simulink model "gradijentni_model"  (R2025a)
settings: Solver=VariableStepAuto  StartTime=0.0  StopTime=100  RelTol=1e-3
values from neighbouring files (symbols this model uses):
  Tf = 1    [mse.m]
settings Model: Creator=neso  LastModifiedBy=Korisnik

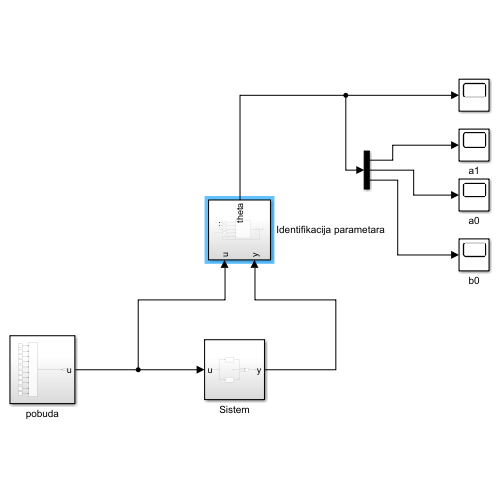
[thumbnail: Simulink's stored preview of the top-level diagram]
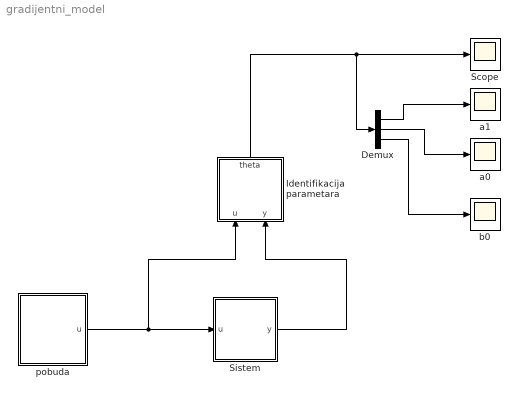
== system gradijentni_model ==
  Demux : Demux  Outputs=3
  Identifikacija parametara : Subsystem
  Scope : Scope
      settings: ActiveDisplayYMinimum=-10.408087644421066  ActiveDisplayYMaximum=16.003973276470475
  Sistem : Subsystem
  a0 : Scope
      settings: ActiveDisplayYMinimum=-8.5109294559908086  ActiveDisplayYMaximum=21.084373521888086  DataLoggingVariableName=ScopeData2
  a1 : Scope
      settings: ActiveDisplayYMinimum=0.935675841003011  ActiveDisplayYMaximum=9.3006227399808985
  b0 : Scope
      settings: ActiveDisplayYMinimum=-8.5109294559908086  ActiveDisplayYMaximum=21.084373521888086  DataLoggingVariableName=ScopeData3
  pobuda : Subsystem
  wires:
  Sistem/1(y) -> Identifikacija parametara/2(y)
  Identifikacija parametara/1(theta) -> Demux/1, Scope/1
  pobuda/1(u) -> Identifikacija parametara/1(u), Sistem/1(u)
  Demux/1 -> a1/1
  Demux/2 -> a0/1
  Demux/3 -> b0/1

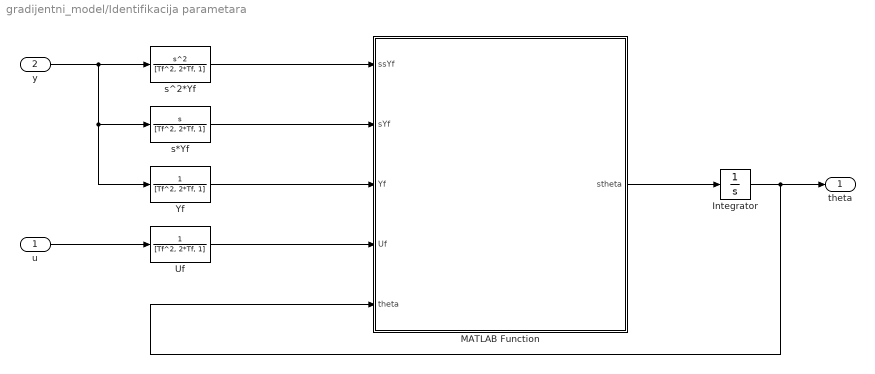
== system gradijentni_model/Identifikacija parametara ==
  u : Inport
  y : Inport  Port=2
  Integrator : Integrator  InitialCondition=[0; 0; 0]
  MATLAB Function : MATLAB Function  TreatAsAtomicUnit=on
  Uf : TransferFcn  Denominator=[Tf^2, 2*Tf, 1]
  Yf : TransferFcn  Denominator=[Tf^2, 2*Tf, 1]
  s*Yf : TransferFcn  Numerator=[1, 0]  Denominator=[Tf^2, 2*Tf, 1]
  s^2*Yf : TransferFcn  Numerator=[1, 0, 0]  Denominator=[Tf^2, 2*Tf, 1]
  theta : Outport
  wires:
  y/1 -> Yf/1, s*Yf/1, s^2*Yf/1
  u/1 -> Uf/1
  s^2*Yf/1 -> MATLAB Function/1(ssYf)
  s*Yf/1 -> MATLAB Function/2(sYf)
  Yf/1 -> MATLAB Function/3(Yf)
  Uf/1 -> MATLAB Function/4(Uf)
  MATLAB Function/1(stheta) -> Integrator/1
  Integrator/1 -> MATLAB Function/5(theta), theta/1

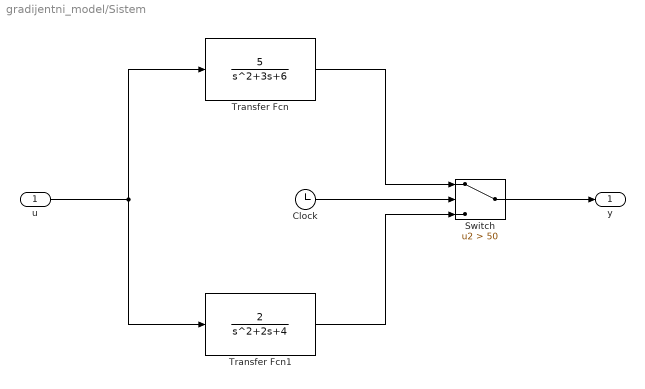
== system gradijentni_model/Sistem ==
  u : Inport
  Clock : Clock
  Switch : Switch  Criteria=u2 > Threshold  Threshold=50  SaturateOnIntegerOverflow=off  InputSameDT=off
  Transfer Fcn : TransferFcn  Numerator=[5]  Denominator=[1, 3, 6]
  Transfer Fcn1 : TransferFcn  Numerator=2  Denominator=[1, 2, 4]
  y : Outport
  wires:
  u/1 -> Transfer Fcn1/1, Transfer Fcn/1
  Transfer Fcn/1 -> Switch/1
  Transfer Fcn1/1 -> Switch/3
  Switch/1 -> y/1
  Clock/1 -> Switch/2

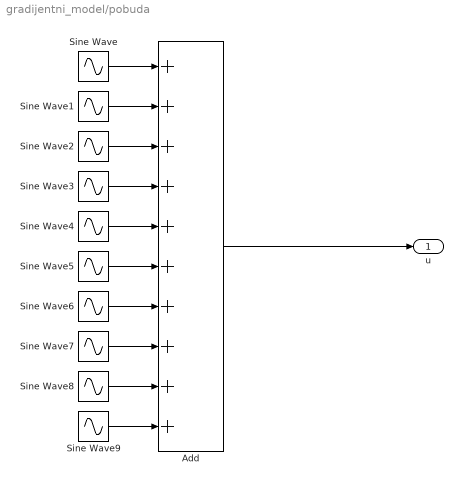
== system gradijentni_model/pobuda ==
  Add : Sum  Inputs=10
  Sine Wave : Sin  SampleTime=0
  Sine Wave1 : Sin  Frequency=2  SampleTime=0
  Sine Wave2 : Sin  Frequency=3  SampleTime=0
  Sine Wave3 : Sin  Frequency=4  SampleTime=0
  Sine Wave4 : Sin  Frequency=5  SampleTime=0
  Sine Wave5 : Sin  Frequency=6  SampleTime=0
  Sine Wave6 : Sin  Frequency=7  SampleTime=0
  Sine Wave7 : Sin  Frequency=8  SampleTime=0
  Sine Wave8 : Sin  Frequency=9  SampleTime=0
  Sine Wave9 : Sin  Frequency=10  SampleTime=0
  u : Outport
  wires:
  Add/1 -> u/1
  Sine Wave/1 -> Add/1
  Sine Wave1/1 -> Add/2
  Sine Wave2/1 -> Add/3
  Sine Wave3/1 -> Add/4
  Sine Wave4/1 -> Add/5
  Sine Wave5/1 -> Add/6
  Sine Wave6/1 -> Add/7
  Sine Wave7/1 -> Add/8
  Sine Wave8/1 -> Add/9
  Sine Wave9/1 -> Add/10

== matlab function gradijentni_model/Identifikacija parametara/MATLAB Function ==
  data: ssYf input; sYf input; Yf input; Uf input; stheta output; theta input
function stheta = fcn(ssYf, sYf, Yf, Uf, theta)
    p = [-sYf; -Yf; Uf];
    eta = ssYf;
    
    G = 2.5 * eye(length(p), length(p));
    stheta = G * p * (eta - p' * theta);
end
